simulink model "ClassD_Analog_Simulink"  (R2026a)
settings: Solver=VariableStepAuto  StopTime=5e-3
settings Model: Creator=Cullum  LastModifiedBy=Cullum

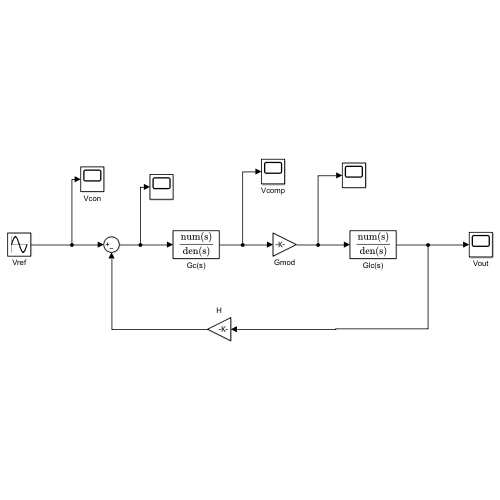
[thumbnail: Simulink's stored preview of the top-level diagram]
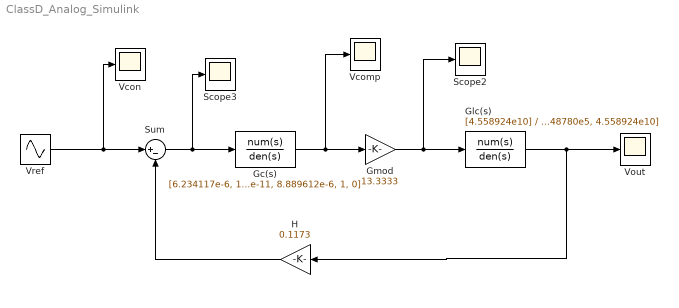
== system ClassD_Analog_Simulink ==
  Gc(s) : TransferFcn  Numerator=[6.234117e-6, 1.558252, 9.708738e4]  Denominator=[1.973233e-11, 8.889612e-6, 1, 0]
  Glc(s) : TransferFcn  Numerator=[4.558924e10]  Denominator=[1, 3.048780e5, 4.558924e10]
  Gmod : Gain  Gain=13.3333
  H : Gain  Gain=0.1173
  Scope2 : Scope
      settings: ActiveDisplayYMinimum=-10.10722279187145  ActiveDisplayYMaximum=10.382818520061747  DataLoggingVariableName=ScopeData3
  Scope3 : Scope
      settings: ActiveDisplayYMinimum=-0.0627887502515101  ActiveDisplayYMaximum=0.049730082191768978  DataLoggingVariableName=ScopeData4
  Sum : Sum  Inputs=|+-
  Vcomp : Scope
      settings: ActiveDisplayYMinimum=-0.75804360449936992  ActiveDisplayYMaximum=0.77871333578797053
  Vcon : Scope
      settings: ActiveDisplayYMinimum=-1.1874999999998457  ActiveDisplayYMaximum=1.1874999999995306  DataLoggingVariableName=ScopeData2
  Vout : Scope
      settings: ActiveDisplayYMinimum=-10.111740584887883  ActiveDisplayYMaximum=10.231055451556021
  Vref : Sin  Amplitude=0.95  Frequency=2*pi*1000  SampleTime=0
  wires:
  Vref/1 -> Vcon/1, Sum/1
  Sum/1 -> Scope3/1, Gc(s)/1
  Gc(s)/1 -> Vcomp/1, Gmod/1
  Gmod/1 -> Scope2/1, Glc(s)/1
  Glc(s)/1 -> Vout/1, H/1
  H/1 -> Sum/2
